simulink model "ControlLane"  (R2024b)
settings: Solver=VariableStepAuto  StartTime=0.0  StopTime=10.0  RelTol=1e-3
settings Model: DataDictionary=Data.sldd  Creator=toma  LastModifiedBy=toma
settings ModelReferenceCC: UpdateModelReferenceTargets=IfOutOfDate
settings ConfigComp: CovBoundaryAbsTol=1.0e-5

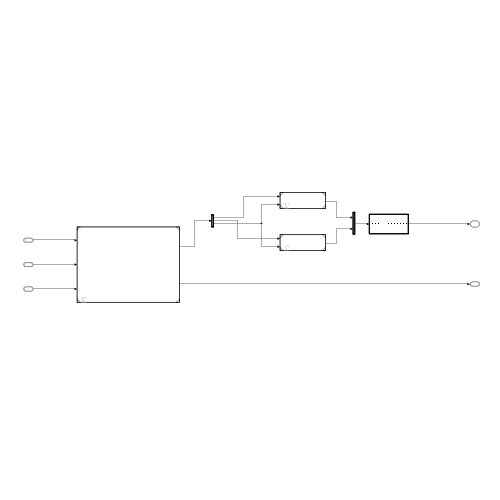
[thumbnail: Simulink's stored preview of the top-level diagram]
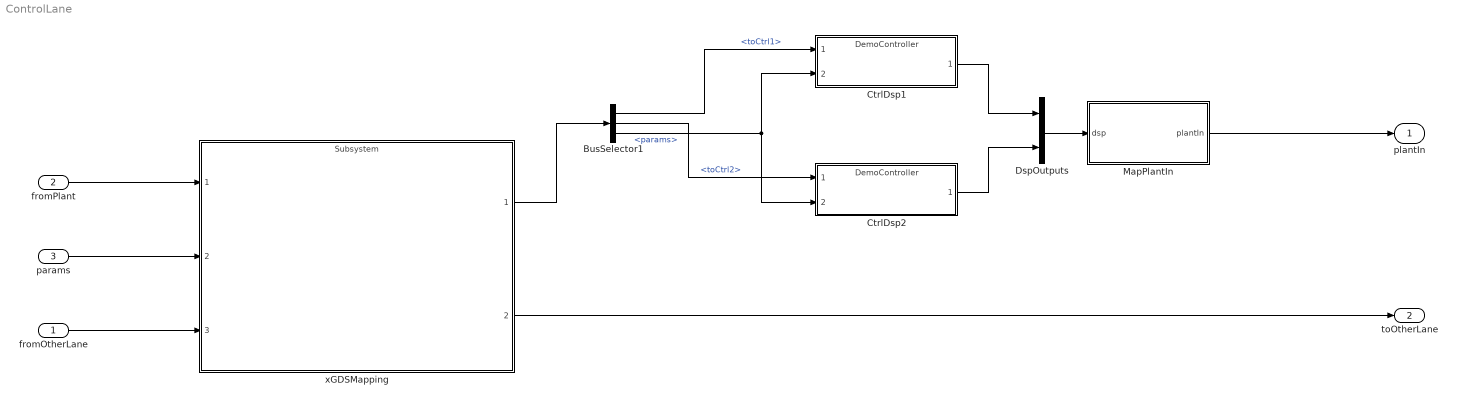
== system ControlLane ==
  fromOtherLane : Inport  OutDataTypeStr=Bus: toCtrl
  fromPlant : Inport  Port=2  OutDataTypeStr=Bus: PlantOut
  params : Inport  Port=3  OutDataTypeStr=Bus: ExtParams
  BusSelector1 : BusSelector  OutputSignals=toCtrl1,toCtrl2,params
  CtrlDsp1 : ModelReference  ModelNameDialog=DemoController  SimulationMode=Normal  ModelReferenceVersion=2.1
  CtrlDsp2 : ModelReference  ModelNameDialog=DemoController  SimulationMode=Normal  ModelReferenceVersion=2.1
  DspOutputs : BusCreator  Inputs=2  OutDataTypeStr=Bus: DspOutputs
  MapPlantIn : MATLAB Function  TreatAsAtomicUnit=on
  xGDSMapping : ModelReference  ModelNameDialog=Subsystem  SimulationMode=Normal  ModelReferenceVersion=1.12
  plantIn : Outport  OutDataTypeStr=Bus: LanePlantIn
  toOtherLane : Outport  Port=2  OutDataTypeStr=Bus: toCtrl
  wires:
  fromPlant/1 -> xGDSMapping/1
  fromOtherLane/1 -> xGDSMapping/3
  xGDSMapping/1 -> BusSelector1/1
  xGDSMapping/2 -> toOtherLane/1
  BusSelector1/1 -> CtrlDsp1/1  "<toCtrl1>"
  BusSelector1/2 -> CtrlDsp2/1  "<toCtrl2>"
  BusSelector1/3 -> CtrlDsp1/2, CtrlDsp2/2  "<params>"
  params/1 -> xGDSMapping/2
  CtrlDsp1/1 -> DspOutputs/1
  CtrlDsp2/1 -> DspOutputs/2
  DspOutputs/1 -> MapPlantIn/1(dsp)
  MapPlantIn/1(plantIn) -> plantIn/1

== matlab function ControlLane/MapPlantIn ==
  data: dsp input Bus: DspOutputs; plantIn output Bus: LanePlantIn
function plantIn = fcn(dsp)

plantIn.pOut.a_p = dsp.ctrlDsp1.a;
plantIn.pOut.a1_p = dsp.ctrlDsp1.a1;
plantIn.pOut.a2_p = dsp.ctrlDsp1.a2;
plantIn.pOut1.a_p = dsp.ctrlDsp2.a;
plantIn.pOut1.a1_p = dsp.ctrlDsp2.a1;
plantIn.pOut1.a2_p = dsp.ctrlDsp2.a2;

end
